simulink model "Tourelle2Axes_Sujet"  (R2021b)
settings: Solver=VariableStepAuto  StartTime=0.0  StopTime=2  RelTol=1e-3
values from neighbouring files (symbols this model uses):
  Jm = 1.8135e-7    (= 1.8135e-07)    [Tourelle2Axes.m]
  Jp = 0.0595e-7    (= 5.95e-09)    [Tourelle2Axes.m]
  Km = 0.019    [Tourelle2Axes.m]
  Lm = 35e-3    (= 0.035)    [Tourelle2Axes.m]
  r = 516.6    [Tourelle2Axes.m]
  Rm = 53    [Tourelle2Axes.m]
libraries: slctrlblks x1
settings Model: Creator=xpess  LastModifiedBy=xavier.pessoles2
settings SolverCC: AlgebraicLoopSolver=TrustRegion
settings DebuggingCC: SFMachineParentedDataDiag=warning

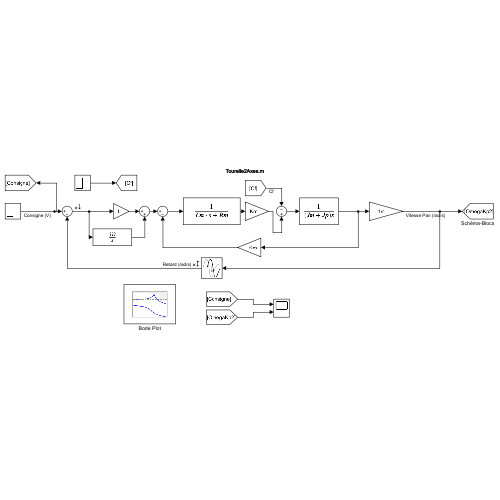
[thumbnail: Simulink's stored preview of the top-level diagram]
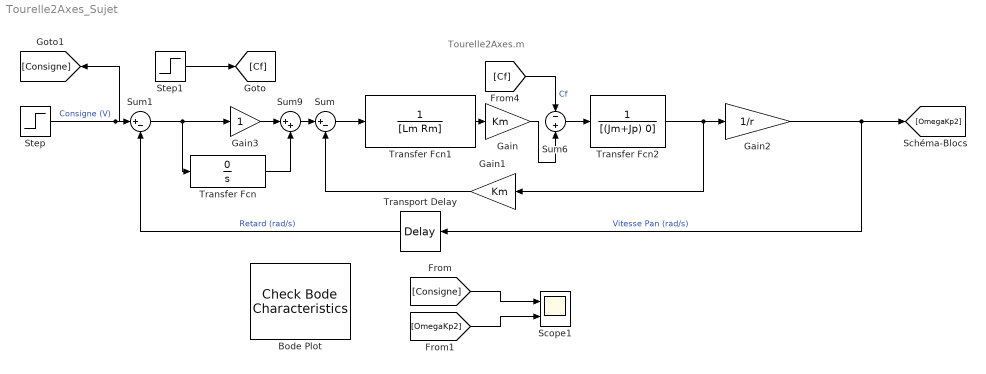
== system Tourelle2Axes_Sujet ==
  note: Tourelle2Axes.m
  Bode Plot : slctrlblks/Model Verification/Check Bode  Characteristics  InstantiateOnLoad=on  SaveOperatingPoints=off  LinearizationIOs={'/Sum1', 1, 'in', 'on', '';'/Transport Delay', 1, 'out', 'on', ''}  LinearizeAt=SnapshotTimes  SnapshotTimes=[0]  TriggerType=rising  SampleTime=auto  RateConversionMethod=zoh  PreWarpFreq=10  UseExactDelayModel=off  UseFullBlockNameLabels=off  UseBusSignalLabels=off  enabled=on  stopWhenAssertionFail=off  export=off  ViewDlgPos=[146.333333333333 41.6666666666667 510 599.333333333333]  OpenViewOnLoad=off  LaunchViewOnOpen=off  FrequencyUnits=rad/s  MagnitudeUnits=dB  PhaseUnits=deg  TimeUnits=seconds  EnableUpperBound=off  UpperBoundFrequencies=[]  UpperBoundMagnitudes=[]  EnableLowerBound=off  LowerBoundFrequencies=[]  LowerBoundMagnitudes=[]
  Gain : Gain  Gain=Km
  Gain1 : Gain  Gain=Km
  Gain2 : Gain  Gain=1/r
  Gain3 : Gain
  Scope1 : Scope  NumInputPorts=2
  Step : Step  Time=0  SampleTime=0
  Step1 : Step  Time=0  After=0.304e-3  SampleTime=0
  Sum : Sum  Inputs=|+-
  Sum1 : Sum  Inputs=|+-
  Sum6 : Sum  Inputs=-|+
  Sum9 : Sum  Inputs=|++
  Transfer Fcn : TransferFcn  Numerator=[0]  Denominator=[1 0]
  Transfer Fcn1 : TransferFcn  Denominator=[Lm Rm]
  Transfer Fcn2 : TransferFcn  Denominator=[(Jm+Jp) 0]
  Transport Delay : TransportDelay  DelayTime=.1
  wires:
  Gain1/1 -> Sum/2
  Gain2/1 -> Transport Delay/1, [OmegaKp2]  "Vitesse Pan (rad/s)"
  Transfer Fcn1/1 -> Gain/1
  Transfer Fcn2/1 -> Gain2/1, Gain1/1
  Sum/1 -> Transfer Fcn1/1
  [Consigne] -> Scope1/1
  [OmegaKp2] -> Scope1/2
  Transport Delay/1 -> Sum1/2  "Retard (rad/s)"
  Sum1/1 -> Transfer Fcn/1, Gain3/1
  Step/1 -> [Consigne], Sum1/1  "Consigne (V)"
  Sum6/1 -> Transfer Fcn2/1
  Gain/1 -> Sum6/2
  [Cf] -> Sum6/1  "Cf"
  Step1/1 -> [Cf]
  Gain3/1 -> Sum9/1
  Sum9/1 -> Sum/1
  Transfer Fcn/1 -> Sum9/2
